simulink model "Sim_Forcing_003h_expe_infra5_full_control2"  (Simulink 7.4)
settings: Solver=FixedStepDiscrete  StartTime=0.0  StopTime=inf  FixedStep=0.004  RelTol=1e-3
undefined symbols (not defined in the file or in its folder): DiscIntNeverNeededParam
libraries: simulink x43, gt_rt_lib x22, xpcutilitieslib x4, xpclib x2, dspswit3 x1
(part 2 of 4)

== system Sim_Forcing_003h_expe_infra5_full_control2/Breaking_Control 20/07/15/Smooth Displacement Second-Order Filter, zeta 0.8 ==
  Step IN Reset on  either : Inport
  T : Inport  Port=2  OutDataType=fixdt(1, 16)  OutScaling=2^0
  (zeta*T_transfer)/pi : Gain  Gain=0.8/pi  ParameterDataType=fixdt(1, 16)  ParameterScaling=2^0  OutDataType=fixdt(1, 16)  OutScaling=2^0
  4*zeta*pi : Gain  Gain=3.2*pi  ParameterDataType=fixdt(1, 16)  ParameterScaling=2^0  OutDataType=fixdt(1, 16)  OutScaling=2^0
  4*zeta*pi/T_transfer /s : DiscreteIntegrator  gainval=1  ExternalReset=either  InitialConditionSource=external  SampleTime=0.004  OutDataType=fixdt(1, 16)  OutScaling=2^0  ICPrevOutput=DiscIntNeverNeededParam  ICPrevScaledInput=DiscIntNeverNeededParam
  Discrete Derivative : simulink/Discrete/Discrete Derivative  SystemSampleTime=-1  gainval=1.0  ICPrevScaledInput=0.0  OutMin=[]  OutMax=[]  OutDataType=fixdt(1, 16)  OutScaling=2^-10  DoSatur=off
  Divide : Product  Inputs=*/  OutDataType=fixdt(1, 16)  OutScaling=2^-10
  Divide1 : Product  Inputs=*/  OutDataType=fixdt(1, 16)  OutScaling=2^-10
  For saving position  and velocity until after switchover : UnitDelay  SampleTime=-1
  Product : Product  OutDataType=fixdt(1, 16)  OutScaling=2^0  RndMeth=Zero
  Sum1 : Sum  Inputs=|+-  OutDataType=fixdt(1, 16)  OutScaling=2^0
  Sum2 : Sum  Inputs=-+|  OutDataType=fixdt(1, 16)  OutScaling=2^0
  pi/(zeta*T_transfer)/s : DiscreteIntegrator  gainval=1  ExternalReset=either  InitialConditionSource=external  SampleTime=0.004  OutDataType=fixdt(1, 16)  OutScaling=2^0  ICPrevOutput=DiscIntNeverNeededParam  ICPrevScaledInput=DiscIntNeverNeededParam
  pi/zeta : Gain  Gain=pi/0.8  ParameterDataType=fixdt(1, 16)  ParameterScaling=2^0  OutDataType=fixdt(1, 16)  OutScaling=2^0
  Out : Outport
  wires:
  Discrete Derivative/1 -> Product/2
  Product/1 -> (zeta*T_transfer)/pi/1
  Divide/1 -> 4*zeta*pi/1
  Divide1/1 -> pi/zeta/1
  pi/zeta/1 -> pi/(zeta*T_transfer)/s/1
  pi/(zeta*T_transfer)/s/1 -> Sum2/1, Out/1, For saving position  and velocity until after switchover/1
  4*zeta*pi/T_transfer /s/1 -> Divide1/1, Sum1/2
  Sum1/1 -> Divide/1
  4*zeta*pi/1 -> 4*zeta*pi/T_transfer /s/1
  T/1 -> [T]
  Step IN Reset on  either/1 -> [Step], Sum2/2
  [Step] -> 4*zeta*pi/T_transfer /s/2
  [Step] -> pi/(zeta*T_transfer)/s/2
  [T] -> Divide/2
  For saving position  and velocity until after switchover/1 -> Discrete Derivative/1, pi/(zeta*T_transfer)/s/3
  [T] -> Product/1
  (zeta*T_transfer)/pi/1 -> 4*zeta*pi/T_transfer /s/3
  [T] -> Divide1/2
  Sum2/1 -> Sum1/1

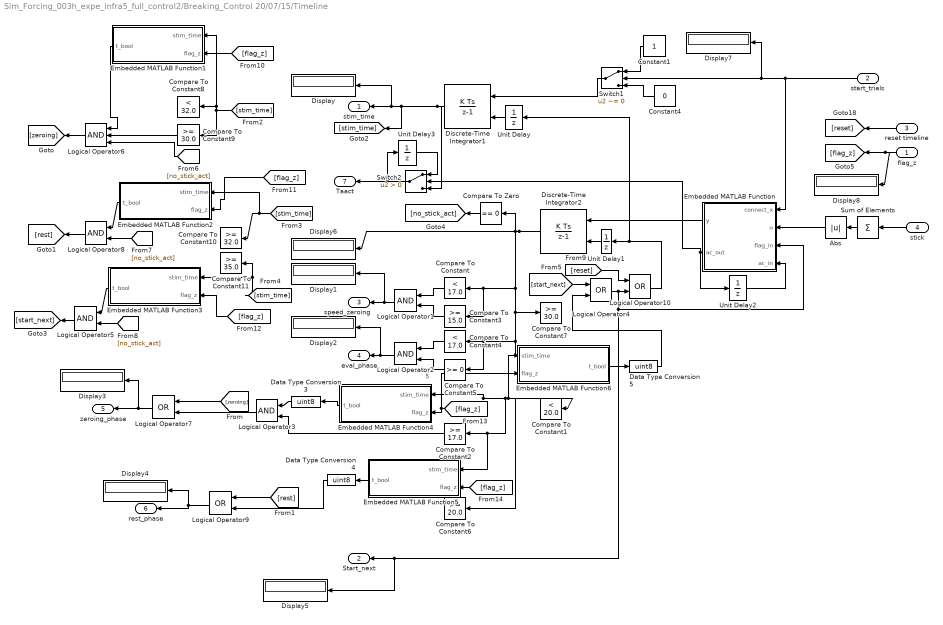
== system Sim_Forcing_003h_expe_infra5_full_control2/Breaking_Control 20/07/15/Timeline ==
  note: 5
  flag_z : Inport  PortDimensions=1
  start_trials : Inport  Port=2  PortDimensions=1
  reset timeline : Inport  Port=3  PortDimensions=1
  stick : Inport  Port=4
  Abs : Abs  OutDataType=fixdt(1, 16)  OutScaling=2^0
  Compare To Constant : simulink/Logic and Bit Operations/Compare To Constant  SystemSampleTime=-1  relop=<  const=17.0  LogicOutDataTypeMode=uint8
  Compare To Constant1 : simulink/Logic and Bit Operations/Compare To Constant  SystemSampleTime=-1  relop=<  const=20.0  LogicOutDataTypeMode=uint8
  Compare To Constant10 : simulink/Logic and Bit Operations/Compare To Constant  SystemSampleTime=-1  relop=>=  const=32.0  LogicOutDataTypeMode=uint8
  Compare To Constant11 : simulink/Logic and Bit Operations/Compare To Constant  SystemSampleTime=-1  relop=>=  const=35.0  LogicOutDataTypeMode=uint8
  Compare To Constant2 : simulink/Logic and Bit Operations/Compare To Constant  SystemSampleTime=-1  relop=>=  const=17.0  LogicOutDataTypeMode=uint8
  Compare To Constant3 : simulink/Logic and Bit Operations/Compare To Constant  SystemSampleTime=-1  relop=>=  const=15.0  LogicOutDataTypeMode=uint8
  Compare To Constant4 : simulink/Logic and Bit Operations/Compare To Constant  SystemSampleTime=-1  relop=<  const=17.0  LogicOutDataTypeMode=uint8
  Compare To Constant5 : simulink/Logic and Bit Operations/Compare To Constant  SystemSampleTime=-1  relop=>=  const=0  LogicOutDataTypeMode=uint8
  Compare To Constant6 : simulink/Logic and Bit Operations/Compare To Constant  SystemSampleTime=-1  relop=>=  const=20.0  LogicOutDataTypeMode=uint8
  Compare To Constant7 : simulink/Logic and Bit Operations/Compare To Constant  SystemSampleTime=-1  relop=>=  const=30.0  LogicOutDataTypeMode=uint8
  Compare To Constant8 : simulink/Logic and Bit Operations/Compare To Constant  SystemSampleTime=-1  relop=<  const=32.0  LogicOutDataTypeMode=uint8
  Compare To Constant9 : simulink/Logic and Bit Operations/Compare To Constant  SystemSampleTime=-1  relop=>=  const=30.0  LogicOutDataTypeMode=uint8
  Compare To Zero : simulink/Logic and Bit Operations/Compare To Zero  SystemSampleTime=-1  relop===  LogicOutDataTypeMode=uint8
  Constant1 : Constant  OutDataType=fixdt(1, 16)  OutScaling=2^0
  Constant4 : Constant  Value=0  OutDataType=fixdt(1, 16)  OutScaling=2^0
  Data Type Conversion3 : DataTypeConversion  OutDataTypeMode=uint8  OutDataType=fixdt(1, 16)  OutScaling=2^0  OutDataTypeStr=uint8
  Data Type Conversion4 : DataTypeConversion  OutDataTypeMode=uint8  OutDataType=fixdt(1, 16)  OutScaling=2^0  OutDataTypeStr=uint8
  Data Type Conversion5 : DataTypeConversion  OutDataTypeMode=uint8  OutDataType=fixdt(1, 16)  OutScaling=2^0  OutDataTypeStr=uint8
  Discrete-Time Integrator1 : DiscreteIntegrator  ExternalReset=rising  SampleTime=0.004  LimitOutput=on  UpperSaturationLimit=60  LowerSaturationLimit=0  ICPrevOutput=DiscIntNeverNeededParam  ICPrevScaledInput=DiscIntNeverNeededParam
  Discrete-Time Integrator2 : DiscreteIntegrator  ExternalReset=rising  SampleTime=0.004  LimitOutput=on  UpperSaturationLimit=40  LowerSaturationLimit=0  ICPrevOutput=DiscIntNeverNeededParam  ICPrevScaledInput=DiscIntNeverNeededParam
  Display{,1..8} (9 alike) : Display
  Embedded MATLAB Function : Stateflow chart
  Embedded MATLAB Function1 : Stateflow chart
  Embedded MATLAB Function2 : Stateflow chart
  Embedded MATLAB Function3 : Stateflow chart
  Embedded MATLAB Function4 : Stateflow chart
  Embedded MATLAB Function5 : Stateflow chart
  Embedded MATLAB Function6 : Stateflow chart
  Logical Operator{1..3,5,8} (5 alike) : Logic  AllPortsSameDT=off  OutDataTypeMode=boolean  LogicDataType=fixdt(0, 8)  OutDataTypeStr=boolean
  Logical Operator{4,7,9..10} (4 alike) : Logic  Operator=OR  AllPortsSameDT=off  OutDataTypeMode=boolean  LogicDataType=fixdt(0, 8)  OutDataTypeStr=boolean
  Logical Operator6 : Logic  Inputs=3  AllPortsSameDT=off  OutDataTypeMode=boolean  LogicDataType=fixdt(0, 8)  OutDataTypeStr=boolean
  Sum of Elements : Sum  Inputs=+  OutDataType=fixdt(1, 16)  OutScaling=2^-10
  Switch1 : Switch  Criteria=u2 ~= 0  Threshold=0.2  OutDataType=fixdt(1, 16)  OutScaling=2^0
  Switch2 : Switch  Criteria=u2 > Threshold  OutDataType=fixdt(1, 16)  OutScaling=2^0
  Unit Delay{,1..3} (4 alike) : UnitDelay  SampleTime=-1
  stim_time : Outport  OutDataType=fixdt(1, 16)  OutScaling=2^0
  Start_next : Outport  Port=2  OutDataType=fixdt(1, 16)  OutScaling=2^0
  speed_zeroing : Outport  Port=3  OutDataType=fixdt(1, 16)  OutScaling=2^0
  eval_phase : Outport  Port=4  OutDataType=fixdt(1, 16)  OutScaling=2^0
  zeroing_phase : Outport  Port=5  OutDataType=fixdt(1, 16)  OutScaling=2^0
  rest_phase : Outport  Port=6  OutDataType=fixdt(1, 16)  OutScaling=2^0
  Taact : Outport  Port=7  OutDataType=fixdt(1, 16)  OutScaling=2^0
  wires:
  Discrete-Time Integrator1/1 -> stim_time/1, Display/1, [stim_time], Switch2/3
  Embedded MATLAB Function/1(y) -> Discrete-Time Integrator2/1
  Discrete-Time Integrator2/1 -> Compare To Constant/1, Compare To Constant3/1, Compare To Constant4/1, Compare To Constant5/1, Compare To Constant1/1, Embedded MATLAB Function4/1(stim_time), Compare To Constant2/1, Embedded MATLAB Function5/1(stim_time), Compare To Constant6/1, Embedded MATLAB Function6/1(stim_time), Compare To Constant7/1, Display6/1, Compare To Zero/1
  Compare To Constant/1 -> Logical Operator1/1
  Compare To Constant3/1 -> Logical Operator1/2
  Logical Operator1/1 -> speed_zeroing/1, Display1/1
  Compare To Constant4/1 -> Logical Operator2/1
  Compare To Constant5/1 -> Logical Operator2/2
  Logical Operator2/1 -> eval_phase/1, Display2/1
  Compare To Constant2/1 -> Logical Operator3/2
  Logical Operator3/1 -> Logical Operator7/2
  Logical Operator4/1 -> Start_next/1, Display5/1, Embedded MATLAB Function/3(flag_in), Logical Operator10/2
  Constant1/1 -> Switch1/1
  Switch1/1 -> Discrete-Time Integrator1/1
  start_trials/1 -> Switch1/2, Display7/1, Embedded MATLAB Function/1(connect_x)
  Constant4/1 -> Switch1/3
  stick/1 -> Sum of Elements/1
  Unit Delay/1 -> Discrete-Time Integrator1/2
  Unit Delay1/1 -> Discrete-Time Integrator2/2
  Sum of Elements/1 -> Abs/1
  Abs/1 -> Embedded MATLAB Function/2(u)
  Embedded MATLAB Function/2(ac_out) -> Unit Delay2/1, Switch2/2
  Unit Delay2/1 -> Embedded MATLAB Function/4(ac_in)
  Compare To Constant9/1 -> Logical Operator6/2
  Logical Operator7/1 -> zeroing_phase/1, Display3/1
  Logical Operator9/1 -> rest_phase/1, Display4/1
  Logical Operator6/1 -> [zeroing]
  [zeroing] -> Logical Operator7/1
  Logical Operator8/1 -> [rest]
  [rest] -> Logical Operator9/1
  [stim_time] -> Compare To Constant9/1, Compare To Constant8/1, Embedded MATLAB Function1/1(stim_time)
  [stim_time] -> Compare To Constant10/1, Embedded MATLAB Function2/1(stim_time)
  [stim_time] -> Compare To Constant11/1, Embedded MATLAB Function3/1(stim_time)
  Logical Operator5/1 -> [start_next]
  [start_next] -> Logical Operator4/1
  Compare To Zero/1 -> [no_stick_act]
  [no_stick_act] -> Logical Operator6/3
  [no_stick_act] -> Logical Operator8/2
  [no_stick_act] -> Logical Operator5/2
  reset timeline/1 -> [reset]
  flag_z/1 -> [flag_z], Display8/1
  [flag_z] -> Embedded MATLAB Function4/2(flag_z), Embedded MATLAB Function6/2(flag_z)
  [flag_z] -> Embedded MATLAB Function5/2(flag_z)
  Embedded MATLAB Function4/1(t_bool) -> Data Type Conversion3/1
  Data Type Conversion3/1 -> Logical Operator3/1
  Embedded MATLAB Function5/1(t_bool) -> Data Type Conversion4/1
  Data Type Conversion4/1 -> Logical Operator9/2
  Embedded MATLAB Function6/1(t_bool) -> Data Type Conversion5/1
  Data Type Conversion5/1 -> Logical Operator4/2
  Switch2/1 -> Taact/1, Unit Delay3/1
  Unit Delay3/1 -> Switch2/1
  [reset] -> Logical Operator10/1
  Logical Operator10/1 -> Unit Delay1/1, Unit Delay/1
  [flag_z] -> Embedded MATLAB Function1/2(flag_z)
  Embedded MATLAB Function1/1(t_bool) -> Logical Operator6/1
  Embedded MATLAB Function2/1(t_bool) -> Logical Operator8/1
  [flag_z] -> Embedded MATLAB Function2/2(flag_z)
  Embedded MATLAB Function3/1(t_bool) -> Logical Operator5/1
  [flag_z] -> Embedded MATLAB Function3/2(flag_z)

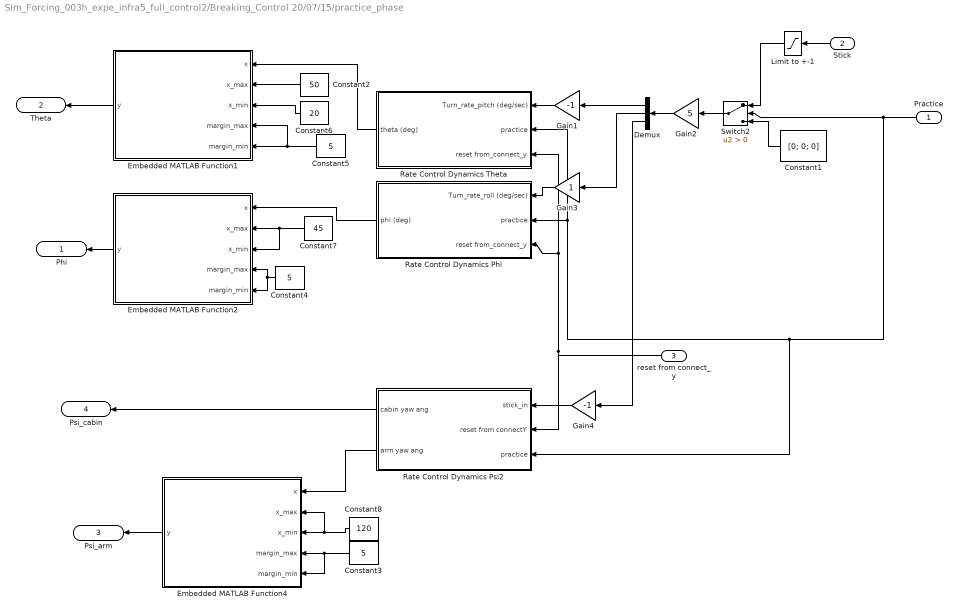
== system Sim_Forcing_003h_expe_infra5_full_control2/Breaking_Control 20/07/15/practice_phase ==
  Practice : Inport  OutDataType=fixdt(1, 16)  OutScaling=2^0
  Stick : Inport  Port=2
  reset from connect_y : Inport  Port=3
  Constant1 : Constant  Value=[0; 0; 0]  OutDataType=fixdt(1, 16)  OutScaling=2^0
  Constant2 : Constant  Value=50  OutDataType=fixdt(1, 16)  OutScaling=2^0
  Constant3 : Constant  Value=5  OutDataType=fixdt(1, 16)  OutScaling=2^0
  Constant4 : Constant  Value=5  OutDataType=fixdt(1, 16)  OutScaling=2^0
  Constant5 : Constant  Value=5  OutDataType=fixdt(1, 16)  OutScaling=2^0
  Constant6 : Constant  Value=20  OutDataType=fixdt(1, 16)  OutScaling=2^0
  Constant7 : Constant  Value=45  OutDataType=fixdt(1, 16)  OutScaling=2^0
  Constant8 : Constant  Value=120  OutDataType=fixdt(1, 16)  OutScaling=2^0
  Demux : Demux  Outputs=3
  Embedded MATLAB Function1 : Stateflow chart
  Embedded MATLAB Function2 : Stateflow chart
  Embedded MATLAB Function4 : Stateflow chart
  Gain1 : Gain  Gain=-1  ParameterDataType=fixdt(1, 16)  ParameterScaling=2^0  OutDataType=fixdt(1, 16)  OutScaling=2^0
  Gain2 : Gain  Gain=5  ParameterDataType=fixdt(1, 16)  ParameterScaling=2^0  OutDataType=fixdt(1, 16)  OutScaling=2^0
  Gain3 : Gain  ParameterDataType=fixdt(1, 16)  ParameterScaling=2^0  OutDataType=fixdt(1, 16)  OutScaling=2^0
  Gain4 : Gain  Gain=-1  ParameterDataType=fixdt(1, 16)  ParameterScaling=2^0  OutDataType=fixdt(1, 16)  OutScaling=2^0
  Limit to +-1 : Saturate  UpperLimit=1  LowerLimit=-1  OutDataType=fixdt(1, 16)  OutScaling=2^0
  Rate Control Dynamics Phi : Subsystem
  Rate Control Dynamics Psi2 : Subsystem
  Rate Control Dynamics Theta : Subsystem
  Switch2 : Switch  Criteria=u2 > Threshold  OutDataType=fixdt(1, 16)  OutScaling=2^0
  Phi : Outport
  Theta : Outport  Port=2
  Psi_arm : Outport  Port=3
  Psi_cabin : Outport  Port=4
  wires:
  Gain2/1 -> Demux/1
  Demux/1 -> Gain1/1
  Demux/2 -> Gain3/1
  Gain1/1 -> Rate Control Dynamics Theta/1(Turn_rate_pitch (deg/sec))
  Switch2/1 -> Gain2/1
  Stick/1 -> Limit to +-1/1
  reset from connect_y/1 -> Rate Control Dynamics Phi/3(reset from_connect_y), Rate Control Dynamics Theta/3(reset from_connect_y), Rate Control Dynamics Psi2/2(reset from connectY)
  Gain3/1 -> Rate Control Dynamics Phi/1(Turn_rate_roll (deg/sec))
  Demux/3 -> Gain4/1
  Practice/1 -> Switch2/2, Rate Control Dynamics Phi/2(practice), Rate Control Dynamics Theta/2(practice), Rate Control Dynamics Psi2/3(practice)
  Limit to +-1/1 -> Switch2/1
  Constant1/1 -> Switch2/3
  Gain4/1 -> Rate Control Dynamics Psi2/1(stick_in)
  Rate Control Dynamics Psi2/1(cabin yaw ang) -> Psi_cabin/1
  Embedded MATLAB Function1/1(y) -> Theta/1
  Constant7/1 -> Embedded MATLAB Function2/2(x_max), Embedded MATLAB Function2/3(x_min)
  Rate Control Dynamics Phi/1(phi (deg)) -> Embedded MATLAB Function2/1(x)
  Embedded MATLAB Function2/1(y) -> Phi/1
  Constant3/1 -> Embedded MATLAB Function4/4(margin_max), Embedded MATLAB Function4/5(margin_min)
  Constant8/1 -> Embedded MATLAB Function4/3(x_min), Embedded MATLAB Function4/2(x_max)
  Embedded MATLAB Function4/1(y) -> Psi_arm/1
  Constant4/1 -> Embedded MATLAB Function2/4(margin_max), Embedded MATLAB Function2/5(margin_min)
  Constant5/1 -> Embedded MATLAB Function1/4(margin_max), Embedded MATLAB Function1/5(margin_min)
  Constant6/1 -> Embedded MATLAB Function1/3(x_min)
  Constant2/1 -> Embedded MATLAB Function1/2(x_max)
  Rate Control Dynamics Theta/1(theta (deg)) -> Embedded MATLAB Function1/1(x)
  Rate Control Dynamics Psi2/2(arm yaw ang) -> Embedded MATLAB Function4/1(x)

== system Sim_Forcing_003h_expe_infra5_full_control2/Breaking_Control 20/07/15/select_ang_speed ==
  Count : Inport  OutDataType=fixdt(1, 16)  OutScaling=2^0
  eval_phase : Inport  Port=2  OutDataType=fixdt(1, 16)  OutScaling=2^0
  Constant : Constant  Value=[0 0 0]  OutDataType=fixdt(1, 16)  OutScaling=2^0
  Embedded MATLAB Function2 : Stateflow chart
  Switch : Switch  Criteria=u2 ~= 0  OutDataType=fixdt(1, 16)  OutScaling=2^0
  Unit Delay : UnitDelay  SampleTime=-1
  Target_ang_speed : Outport
  mask : Outport  Port=2
  vis_cond : Outport  Port=3
  flag_out : Outport  Port=4
  eof : Outport  Port=5
  wires:
  Count/1 -> Embedded MATLAB Function2/1(count)
  eval_phase/1 -> Switch/2
  Embedded MATLAB Function2/1(target_ang_speed) -> Switch/3, Target_ang_speed/1
  Constant/1 -> Switch/1
  Embedded MATLAB Function2/2(mask) -> mask/1
  Embedded MATLAB Function2/3(vis_cond) -> vis_cond/1
  Embedded MATLAB Function2/4(flag_out) -> flag_out/1
  Embedded MATLAB Function2/5(endOffile_out) -> Unit Delay/1, eof/1
  Unit Delay/1 -> Embedded MATLAB Function2/2(endOffile_in)

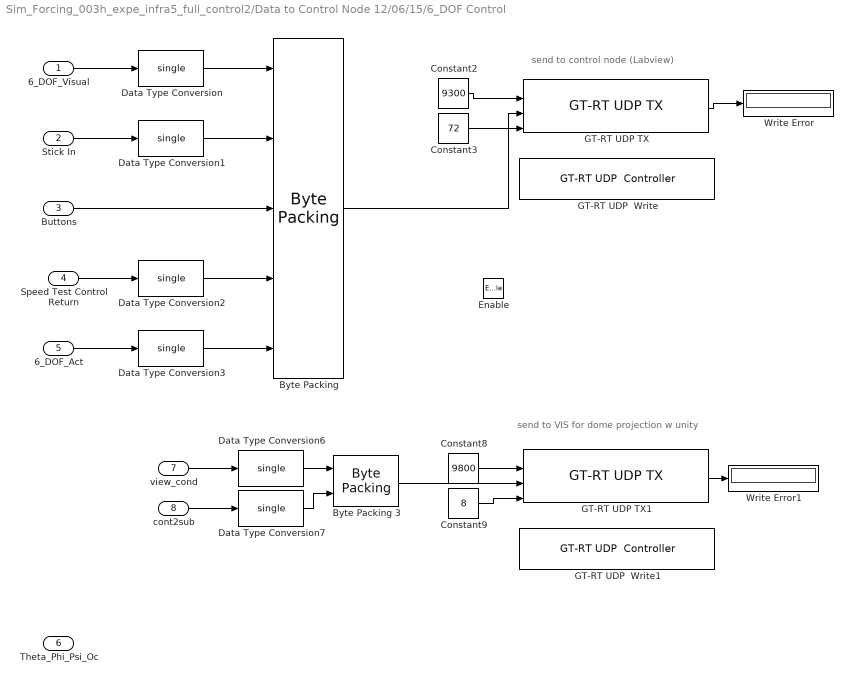
== system Sim_Forcing_003h_expe_infra5_full_control2/Data to Control Node 12/06/15/6_DOF Control ==
  note: send to control node (Labview)
  note: send to VIS for dome projection w unity
  6_DOF_Visual : Inport
  Stick In : Inport  Port=2
  Buttons : Inport  Port=3
  Speed Test Control Return : Inport  Port=4
  6_DOF_Act : Inport  Port=5
  Theta_Phi_Psi_Oc : Inport  Port=6
  view_cond : Inport  Port=7
  cont2sub : Inport  Port=8
  Enable : EnablePort
  "Byte Packing " : xpcutilitieslib/Byte Packing   MaskPackedDataType=uint8  MaskUnpackedDataTypes={'single','single','uint8','single','single'}  MaskAlignment=1
  Byte Packing 3 : xpcutilitieslib/Byte Packing   MaskPackedDataType=uint8  MaskUnpackedDataTypes={'single','single'}  MaskAlignment=1
  Constant2 : Constant  Value=9300  OutDataTypeMode=uint16  OutDataType=fixdt(1, 16)  OutScaling=2^0  OutDataTypeStr=uint16
  Constant3 : Constant  Value=72  OutDataTypeMode=uint32  OutDataType=fixdt(1, 16)  OutScaling=2^0  OutDataTypeStr=uint32
  Constant8 : Constant  Value=9800  OutDataTypeMode=uint16  OutDataType=fixdt(1, 16)  OutScaling=2^0  OutDataTypeStr=uint16
  Constant9 : Constant  Value=8  OutDataTypeMode=uint32  OutDataType=fixdt(1, 16)  OutScaling=2^0  OutDataTypeStr=uint32
  Data Type Conversion{,1..3,6..7} (6 alike) : DataTypeConversion  OutDataTypeMode=single  OutDataType=fixdt(1, 16)  OutScaling=2^0  OutDataTypeStr=single
  GT-RT UDP  Write : gt_rt_lib/GT-RT UDP  Controller  uri='gtp://localhost/udp?port=9300'
  GT-RT UDP  Write1 : gt_rt_lib/GT-RT UDP  Controller  uri='gtp://localhost/udp?port=9800'
  GT-RT UDP TX : gt_rt_lib/GT-RT UDP TX  uri='gtp://localhost/udp?port=9300'  hostname='192.168.102.75'
  GT-RT UDP TX1 : gt_rt_lib/GT-RT UDP TX  uri='gtp://localhost/udp?port=9800'  hostname='192.168.102.13'
  Write Error : Display
  Write Error1 : Display
  wires:
  Constant2/1 -> GT-RT UDP TX/2
  Constant3/1 -> GT-RT UDP TX/4
  GT-RT UDP TX/1 -> Write Error/1
  Data Type Conversion/1 -> "Byte Packing "/1
  "Byte Packing "/1 -> GT-RT UDP TX/3
  Stick In/1 -> Data Type Conversion1/1
  Data Type Conversion1/1 -> "Byte Packing "/2
  Buttons/1 -> "Byte Packing "/3
  Speed Test Control Return/1 -> Data Type Conversion2/1
  Data Type Conversion2/1 -> "Byte Packing "/4
  6_DOF_Act/1 -> Data Type Conversion3/1
  Data Type Conversion3/1 -> "Byte Packing "/5
  GT-RT UDP TX1/1 -> Write Error1/1
  6_DOF_Visual/1 -> Data Type Conversion/1
  Constant8/1 -> GT-RT UDP TX1/2
  Constant9/1 -> GT-RT UDP TX1/4
  Byte Packing 3/1 -> GT-RT UDP TX1/3
  view_cond/1 -> Data Type Conversion6/1
  Data Type Conversion6/1 -> Byte Packing 3/1
  cont2sub/1 -> Data Type Conversion7/1
  Data Type Conversion7/1 -> Byte Packing 3/2

== system Sim_Forcing_003h_expe_infra5_full_control2/Data to Control Node 12/06/15/Interaction device from VIS (Stick)  ==
  Display2 : Display
  Display4 : Display
  Display5 : Display
  Error : Display
  GT-RT UDP  Read : gt_rt_lib/GT-RT UDP  Controller  uri='gtp://localhost/udp?port=9600'
  GT-RT UDP RX : gt_rt_lib/GT-RT UDP RX  uri='gtp://localhost/udp?port=9600'  receive_buffer_size=28  timeout=0  sample_time=0.004
  Terminator : Terminator
  Unpack : xpclib/UDP/Unpack  dimensions={3,8,1,1}  datatypes={'single','uint8','single','single'}  byteAlign=1
  Stick Out : Outport  OutDataType=fixdt(1, 16)  OutScaling=2^0
  Buttons : Outport  Port=2  OutDataType=fixdt(1, 16)  OutScaling=2^0
  Speed_Test_VIS_Send : Outport  Port=3  OutDataType=fixdt(1, 16)  OutScaling=2^0
  for_delay_calc : Outport  Port=4  OutDataType=fixdt(1, 16)  OutScaling=2^0
  wires:
  GT-RT UDP RX/2 -> Display2/1
  GT-RT UDP RX/6 -> Error/1
  GT-RT UDP RX/5 -> Display4/1
  GT-RT UDP RX/4 -> Display5/1
  GT-RT UDP RX/1 -> Unpack/1
  GT-RT UDP RX/3 -> Terminator/1
  Unpack/1 -> Stick Out/1
  Unpack/2 -> Buttons/1
  Unpack/3 -> Speed_Test_VIS_Send/1
  Unpack/4 -> for_delay_calc/1

== system Sim_Forcing_003h_expe_infra5_full_control2/Handshake CAN/If Action Subsystem ==
  Action Port : ActionPort
  GT-RT CAN TX : gt_rt_lib/GT-RT CAN TX  uri='gt_rt_dev://localhost/dev/can0#0'  mff=MFF_11_DAT
  TX CAN ID1 : Constant  Value=hex2dec('100')  OutDataTypeMode=uint32  OutDataType=sfix(16)  OutScaling=2^0  OutDataTypeStr=uint32
  TX Data : Constant  OutDataTypeMode=uint8  OutDataType=sfix(16)  OutScaling=2^0  OutDataTypeStr=uint8
  wires:
  TX CAN ID1/1 -> GT-RT CAN TX/1
  TX Data/1 -> GT-RT CAN TX/2

== system Sim_Forcing_003h_expe_infra5_full_control2/Handshake CAN/If Action Subsystem1 ==
  Action Port : ActionPort  ActionType=then
  GT-RT CAN TX : gt_rt_lib/GT-RT CAN TX  uri='gt_rt_dev://localhost/dev/can0#0'  mff=MFF_11_DAT
  TX CAN ID1 : Constant  Value=hex2dec('100')  OutDataTypeMode=uint32  OutDataType=sfix(16)  OutScaling=2^0  OutDataTypeStr=uint32
  TX Data : Constant  OutDataTypeMode=uint8  OutDataType=sfix(16)  OutScaling=2^0  OutDataTypeStr=uint8
  wires:
  TX CAN ID1/1 -> GT-RT CAN TX/1
  TX Data/1 -> GT-RT CAN TX/2

== system Sim_Forcing_003h_expe_infra5_full_control2/Joint Controller (May 7, 2015)1/Forward Kinematics ==
  J_ANG_ACT : Inport
  Data Type Conversion4 : DataTypeConversion  OutDataTypeMode=double  OutDataType=fixdt(1, 16)  OutScaling=2^0  OutDataTypeStr=double
  Demux1 : Demux  Outputs=[3,1,1,1]
  Embedded MATLAB Function : Stateflow chart
  KUKA2NED : Subsystem
  Mux : Mux  Inputs=3
  6-DOF_ACT : Outport
  roll_pitch_yaw_act : Outport  Port=2
  wires:
  KUKA2NED/1(NED) -> Embedded MATLAB Function/1(vec)
  Embedded MATLAB Function/1(out) -> 6-DOF_ACT/1, Data Type Conversion4/1
  J_ANG_ACT/1 -> KUKA2NED/1(KUKA)
  Demux1/3 -> Mux/2
  Demux1/2 -> Mux/1
  Mux/1 -> roll_pitch_yaw_act/1
  Data Type Conversion4/1 -> Demux1/1
  Demux1/4 -> Mux/3

== system Sim_Forcing_003h_expe_infra5_full_control2/Joint Controller (May 7, 2015)1/Increments ==
  J_ANG : Inport
  Sum6 : Sum  Inputs=|+-  OutDataType=fixdt(1, 16)  OutScaling=2^0
  Unit Delay6 : UnitDelay  X0=[0 50 -68 0 18 0]'  SampleTime=-1
  J_ANG_INC : Outport
  wires:
  Unit Delay6/1 -> Sum6/2
  J_ANG/1 -> Unit Delay6/1, Sum6/1
  Sum6/1 -> J_ANG_INC/1

== system Sim_Forcing_003h_expe_infra5_full_control2/Joint Controller (May 7, 2015)1/Inverse Kinematics May 6, 2015 ==
  note: Delay of 0.004s to initialize the currect step with the value of J_ANG of the previous loop
  6-DOF : Inport  OutDataType=fixdt(1, 16)  OutScaling=2^0
  Activate_full_inverse : Inport  Port=2  OutDataType=fixdt(1, 16)  OutScaling=2^0
  6_DOF_ACT : Inport  Port=3  OutDataType=fixdt(1, 16)  OutScaling=2^0
  Constant : Constant  OutDataType=fixdt(1, 16)  OutScaling=2^0
  Demux : Demux  Outputs=[6 1]
  Ground : Ground
  Inverse Kinematics : Subsystem
  Mux : Mux  Inputs=2
  NED2KUKA : Subsystem
  Scope1 : Scope
      settings: YMin=-50  YMax=70  SaveName=ScopeData4
  Simplified Inverse Kinematics : Subsystem
  Starting Joint Angles KUKA : Constant  Value=[0 -50 68 0 -18 15.89]'  OutDataType=fixdt(1, 16)  OutScaling=2^0
  Starting Joint Angles NED : Constant  Value=[0 50 -68 0 18 0]'  OutDataType=fixdt(1, 16)  OutScaling=2^0
  Switch : Switch  Criteria=u2 > Threshold  OutDataType=fixdt(1, 16)  OutScaling=2^0
  Switch1 : Switch  Criteria=u2 > Threshold  OutDataType=fixdt(1, 16)  OutScaling=2^0
  Unit Delay : UnitDelay  X0=[0 50 -68 0 18 0]'  SampleTime=-1
  J_ANG : Outport  OutDataType=fixdt(1, 16)  OutScaling=2^0
  N : Outport  Port=2  OutDataType=fixdt(1, 16)  OutScaling=2^0
  wires:
  NED2KUKA/1(KUKA) -> Scope1/1, J_ANG/1
  6-DOF/1 -> Mux/1
  Unit Delay/1 -> Mux/2
  Demux/1 -> NED2KUKA/1(NED), Unit Delay/1
  Demux/2 -> N/1
  Simplified Inverse Kinematics/1(out) -> Switch/1
  Inverse Kinematics/1(out) -> Switch/3
  Switch/1 -> Demux/1
  Mux/1 -> Inverse Kinematics/1(vec), Simplified Inverse Kinematics/2(vec)
  Activate_full_inverse/1 -> Inverse Kinematics/2(Activate full inverse), Switch1/2
  Ground/1 -> Switch1/1
  Switch1/1 -> Simplified Inverse Kinematics/1(activate simplified), Switch/2
  Constant/1 -> Switch1/3
  6_DOF_ACT/1 -> Inverse Kinematics/3(6_DOF_ACT)

== system Sim_Forcing_003h_expe_infra5_full_control2/Joint Controller (May 7, 2015)1/Subtract psi offset ==
  Psi_Offset : Inport
  J_ANG_ACT : Inport  Port=2
  Data Type Conversion : DataTypeConversion  OutDataTypeMode=double  OutDataType=fixdt(1, 16)  OutScaling=2^0  OutDataTypeStr=double
  Demux1 : Demux  Outputs=[1,5]
  Mux1 : Mux  Inputs=[1,5]
  Sum3 : Sum  Inputs=-+|  OutDataType=fixdt(1, 16)  OutScaling=2^0
  out : Outport
  wires:
  Demux1/1 -> Sum3/2
  Sum3/1 -> Mux1/1
  Demux1/2 -> Mux1/2
  J_ANG_ACT/1 -> Data Type Conversion/1
  Mux1/1 -> out/1
  Data Type Conversion/1 -> Demux1/1
  Psi_Offset/1 -> Sum3/1

== system Sim_Forcing_003h_expe_infra5_full_control2/BEC (May 7, 2015)/CAN Receive/Convert 4*uni8 to int ==
  byte0 : Inport
  byte1 : Inport  Port=2
  byte2 : Inport  Port=3
  byte3 : Inport  Port=4
  Add : Sum  Inputs=++++  OutDataTypeMode=int32  OutDataType=fixdt(1, 16)  OutScaling=2^-10  OutDataTypeStr=int32
  Gain2 : Gain  Gain=256  ParameterDataType=fixdt(1, 16)  ParameterScaling=2^0  OutDataType=fixdt(1, 16)  OutScaling=2^0
  Gain3 : Gain  Gain=2^16  ParameterDataType=fixdt(1, 16)  ParameterScaling=2^0  OutDataType=fixdt(1, 16)  OutScaling=2^0
  Gain4 : Gain  Gain=2^24  ParameterDataType=fixdt(1, 16)  ParameterScaling=2^0  OutDataType=fixdt(1, 16)  OutScaling=2^0
  int : Outport
  wires:
  Gain2/1 -> Add/2
  Gain3/1 -> Add/3
  byte0/1 -> Add/1
  Add/1 -> int/1
  byte1/1 -> Gain2/1
  byte2/1 -> Gain3/1
  byte3/1 -> Gain4/1
  Gain4/1 -> Add/4

== system Sim_Forcing_003h_expe_infra5_full_control2/BEC (May 7, 2015)/CAN Receive/Convert 4*uni8 to int1 ==
  byte0 : Inport
  byte1 : Inport  Port=2
  byte2 : Inport  Port=3
  byte3 : Inport  Port=4
  Add : Sum  Inputs=++++  OutDataTypeMode=int32  OutDataType=fixdt(1, 16)  OutScaling=2^-10  OutDataTypeStr=int32
  Gain2 : Gain  Gain=256  ParameterDataType=fixdt(1, 16)  ParameterScaling=2^0  OutDataType=fixdt(1, 16)  OutScaling=2^0
  Gain3 : Gain  Gain=2^16  ParameterDataType=fixdt(1, 16)  ParameterScaling=2^0  OutDataType=fixdt(1, 16)  OutScaling=2^0
  Gain4 : Gain  Gain=2^24  ParameterDataType=fixdt(1, 16)  ParameterScaling=2^0  OutDataType=fixdt(1, 16)  OutScaling=2^0
  int : Outport
  wires:
  Gain4/1 -> Add/4
  byte3/1 -> Gain4/1
  byte2/1 -> Gain3/1
  byte1/1 -> Gain2/1
  Add/1 -> int/1
  byte0/1 -> Add/1
  Gain3/1 -> Add/3
  Gain2/1 -> Add/2

== system Sim_Forcing_003h_expe_infra5_full_control2/BEC (May 7, 2015)/CAN Receive/Convert 4*uni8 to int2 ==
  byte0 : Inport
  byte1 : Inport  Port=2
  byte2 : Inport  Port=3
  byte3 : Inport  Port=4
  Add : Sum  Inputs=++++  OutDataTypeMode=int32  OutDataType=fixdt(1, 16)  OutScaling=2^-10  OutDataTypeStr=int32
  Gain2 : Gain  Gain=256  ParameterDataType=fixdt(1, 16)  ParameterScaling=2^0  OutDataType=fixdt(1, 16)  OutScaling=2^0
  Gain3 : Gain  Gain=2^16  ParameterDataType=fixdt(1, 16)  ParameterScaling=2^0  OutDataType=fixdt(1, 16)  OutScaling=2^0
  Gain4 : Gain  Gain=2^24  ParameterDataType=fixdt(1, 16)  ParameterScaling=2^0  OutDataType=fixdt(1, 16)  OutScaling=2^0
  int : Outport
  wires:
  Gain2/1 -> Add/2
  Gain3/1 -> Add/3
  byte0/1 -> Add/1
  Add/1 -> int/1
  byte1/1 -> Gain2/1
  byte2/1 -> Gain3/1
  byte3/1 -> Gain4/1
  Gain4/1 -> Add/4

== system Sim_Forcing_003h_expe_infra5_full_control2/BEC (May 7, 2015)/CAN Receive/Convert 4*uni8 to int3 ==
  byte0 : Inport
  byte1 : Inport  Port=2
  byte2 : Inport  Port=3
  byte3 : Inport  Port=4
  Add : Sum  Inputs=++++  OutDataTypeMode=int32  OutDataType=fixdt(1, 16)  OutScaling=2^-10  OutDataTypeStr=int32
  Gain2 : Gain  Gain=256  ParameterDataType=fixdt(1, 16)  ParameterScaling=2^0  OutDataType=fixdt(1, 16)  OutScaling=2^0
  Gain3 : Gain  Gain=2^16  ParameterDataType=fixdt(1, 16)  ParameterScaling=2^0  OutDataType=fixdt(1, 16)  OutScaling=2^0
  Gain4 : Gain  Gain=2^24  ParameterDataType=fixdt(1, 16)  ParameterScaling=2^0  OutDataType=fixdt(1, 16)  OutScaling=2^0
  int : Outport
  wires:
  Gain4/1 -> Add/4
  byte3/1 -> Gain4/1
  byte2/1 -> Gain3/1
  byte1/1 -> Gain2/1
  Add/1 -> int/1
  byte0/1 -> Add/1
  Gain3/1 -> Add/3
  Gain2/1 -> Add/2

== system Sim_Forcing_003h_expe_infra5_full_control2/BEC (May 7, 2015)/CAN Receive/Convert 4*uni8 to int4 ==
  byte0 : Inport
  byte1 : Inport  Port=2
  byte2 : Inport  Port=3
  byte3 : Inport  Port=4
  Add : Sum  Inputs=++++  OutDataTypeMode=int32  OutDataType=fixdt(1, 16)  OutScaling=2^-10  OutDataTypeStr=int32
  Gain2 : Gain  Gain=256  ParameterDataType=fixdt(1, 16)  ParameterScaling=2^0  OutDataType=fixdt(1, 16)  OutScaling=2^0
  Gain3 : Gain  Gain=2^16  ParameterDataType=fixdt(1, 16)  ParameterScaling=2^0  OutDataType=fixdt(1, 16)  OutScaling=2^0
  Gain4 : Gain  Gain=2^24  ParameterDataType=fixdt(1, 16)  ParameterScaling=2^0  OutDataType=fixdt(1, 16)  OutScaling=2^0
  int : Outport
  wires:
  Gain2/1 -> Add/2
  Gain3/1 -> Add/3
  byte0/1 -> Add/1
  Add/1 -> int/1
  byte1/1 -> Gain2/1
  byte2/1 -> Gain3/1
  byte3/1 -> Gain4/1
  Gain4/1 -> Add/4

== system Sim_Forcing_003h_expe_infra5_full_control2/BEC (May 7, 2015)/CAN Receive/Convert 4*uni8 to int5 ==
  byte0 : Inport
  byte1 : Inport  Port=2
  byte2 : Inport  Port=3
  byte3 : Inport  Port=4
  Add : Sum  Inputs=++++  OutDataTypeMode=int32  OutDataType=fixdt(1, 16)  OutScaling=2^-10  OutDataTypeStr=int32
  Gain2 : Gain  Gain=256  ParameterDataType=fixdt(1, 16)  ParameterScaling=2^0  OutDataType=fixdt(1, 16)  OutScaling=2^0
  Gain3 : Gain  Gain=2^16  ParameterDataType=fixdt(1, 16)  ParameterScaling=2^0  OutDataType=fixdt(1, 16)  OutScaling=2^0
  Gain4 : Gain  Gain=2^24  ParameterDataType=fixdt(1, 16)  ParameterScaling=2^0  OutDataType=fixdt(1, 16)  OutScaling=2^0
  int : Outport
  wires:
  Gain4/1 -> Add/4
  byte3/1 -> Gain4/1
  byte2/1 -> Gain3/1
  byte1/1 -> Gain2/1
  Add/1 -> int/1
  byte0/1 -> Add/1
  Gain3/1 -> Add/3
  Gain2/1 -> Add/2

== system Sim_Forcing_003h_expe_infra5_full_control2/BEC (May 7, 2015)/CAN Send/If Action Subsystem1 ==
  In1 : Inport  OutDataType=fixdt(1, 16)  OutScaling=2^0
  In2 : Inport  Port=2  OutDataType=fixdt(1, 16)  OutScaling=2^0
  In3 : Inport  Port=3  OutDataType=fixdt(1, 16)  OutScaling=2^0
  In4 : Inport  Port=4  OutDataType=fixdt(1, 16)  OutScaling=2^0
  In5 : Inport  Port=5  OutDataType=fixdt(1, 16)  OutScaling=2^0
  In6 : Inport  Port=6  OutDataType=fixdt(1, 16)  OutScaling=2^0
  Action Port : ActionPort  ActionType=then
  "Convert int to 4*uni8 " : Subsystem
  Convert int to 4*uni8 1 : Subsystem
  Convert int to 4*uni8 2 : Subsystem
  Convert int to 4*uni8 3 : Subsystem
  Convert int to 4*uni8 4 : Subsystem
  Convert int to 4*uni8 5 : Subsystem
  GT-RT CAN TX : gt_rt_lib/GT-RT CAN TX  uri='gt_rt_dev://localhost/dev/can0#0'  mff=MFF_11_DAT
  GT-RT CAN TX1 : gt_rt_lib/GT-RT CAN TX  uri='gt_rt_dev://localhost/dev/can0#0'  mff=MFF_11_DAT
  GT-RT CAN TX2 : gt_rt_lib/GT-RT CAN TX  uri='gt_rt_dev://localhost/dev/can0#0'  mff=MFF_11_DAT
  Mux : Mux  Inputs=2
  Mux1 : Mux  Inputs=2
  Mux2 : Mux  Inputs=2
  TX CAN ID1 : Constant  Value=hex2dec('101')  OutDataTypeMode=uint32  OutDataType=sfix(16)  OutScaling=2^0  OutDataTypeStr=uint32
  TX CAN ID2 : Constant  Value=hex2dec('102')  OutDataTypeMode=uint32  OutDataType=sfix(16)  OutScaling=2^0  OutDataTypeStr=uint32
  TX CAN ID3 : Constant  Value=hex2dec('103')  OutDataTypeMode=uint32  OutDataType=sfix(16)  OutScaling=2^0  OutDataTypeStr=uint32
  wires:
  In1/1 -> "Convert int to 4*uni8 "/1(in)
  In2/1 -> Convert int to 4*uni8 1/1(in)
  In3/1 -> Convert int to 4*uni8 2/1(in)
  In4/1 -> Convert int to 4*uni8 3/1(in)
  In5/1 -> Convert int to 4*uni8 4/1(in)
  In6/1 -> Convert int to 4*uni8 5/1(in)
  Mux2/1 -> GT-RT CAN TX2/2
  Convert int to 4*uni8 5/1(out) -> Mux2/2
  Convert int to 4*uni8 4/1(out) -> Mux2/1
  Mux1/1 -> GT-RT CAN TX1/2
  Convert int to 4*uni8 3/1(out) -> Mux1/2
  Convert int to 4*uni8 2/1(out) -> Mux1/1
  Mux/1 -> GT-RT CAN TX/2
  Convert int to 4*uni8 1/1(out) -> Mux/2
  "Convert int to 4*uni8 "/1(out) -> Mux/1
  TX CAN ID3/1 -> GT-RT CAN TX2/1
  TX CAN ID2/1 -> GT-RT CAN TX1/1
  TX CAN ID1/1 -> GT-RT CAN TX/1

== system Sim_Forcing_003h_expe_infra5_full_control2/BEC (May 7, 2015)/Software limit switches/Subsystem ==
  In1 : Inport
  act : Inport  Port=2
  Abs1 : Abs  OutDataType=fixdt(1, 16)  OutScaling=2^0
  Abs2 : Abs  OutDataType=fixdt(1, 16)  OutScaling=2^0
  Add1 : Sum  Inputs=+-  OutDataType=fixdt(1, 16)  OutScaling=2^-10
  Add2 : Sum  Inputs=-+  OutDataType=fixdt(1, 16)  OutScaling=2^-10
  Display : Display
  Display2 : Display
  If Action Subsystem : Subsystem  TreatAsAtomicUnit=on
  If Action Subsystem1 : Subsystem  TreatAsAtomicUnit=on
  If2 : If
  NSEA1 : Constant  Value=-160  OutDataType=fixdt(1, 16)  OutScaling=2^0
  PSEA1 : Constant  Value=160  OutDataType=fixdt(1, 16)  OutScaling=2^0
  Switch : Switch  Criteria=u2 > Threshold  OutDataType=fixdt(1, 16)  OutScaling=2^0
  Switch1 : Switch  Criteria=u2 ~= 0  OutDataType=fixdt(1, 16)  OutScaling=2^0
  Out1 : Outport
  wires:
  If Action Subsystem1/1(Out1) -> Switch/3
  If Action Subsystem/1(Out1) -> Display/1, Switch/1
  Abs1/1 -> If Action Subsystem1/2(dif)
  If2/2 -> If Action Subsystem1/Action
  If2/1 -> If Action Subsystem/Action
  In1/1 -> If2/1, If Action Subsystem/2(Inc), If Action Subsystem1/1(Inc), Switch/2, Switch1/2, Switch1/3
  Abs2/1 -> If Action Subsystem/1(dif)
  NSEA1/1 -> Add1/2
  PSEA1/1 -> Add2/1
  Add1/1 -> Abs1/1
  Add2/1 -> Abs2/1
  Switch/1 -> Switch1/1
  Switch1/1 -> Out1/1, Display2/1
  act/1 -> Add1/1, Add2/2

== system Sim_Forcing_003h_expe_infra5_full_control2/BEC (May 7, 2015)/Software limit switches/Subsystem1 ==
  In1 : Inport
  act : Inport  Port=2
  Abs1 : Abs  OutDataType=fixdt(1, 16)  OutScaling=2^0
  Abs2 : Abs  OutDataType=fixdt(1, 16)  OutScaling=2^0
  Add1 : Sum  Inputs=+-  OutDataType=fixdt(1, 16)  OutScaling=2^-10
  Add2 : Sum  Inputs=-+  OutDataType=fixdt(1, 16)  OutScaling=2^-10
  If Action Subsystem : Subsystem  TreatAsAtomicUnit=on
  If Action Subsystem1 : Subsystem  TreatAsAtomicUnit=on
  If2 : If
  NSEA1 : Constant  Value=-130  OutDataType=fixdt(1, 16)  OutScaling=2^0
  PSEA1 : Constant  Value=20  OutDataType=fixdt(1, 16)  OutScaling=2^0
  Switch : Switch  OutDataType=fixdt(1, 16)  OutScaling=2^0
  Switch1 : Switch  Criteria=u2 ~= 0  OutDataType=fixdt(1, 16)  OutScaling=2^0
  Out1 : Outport
  wires:
  act/1 -> Add1/1, Add2/2
  Add2/1 -> Abs2/1
  Add1/1 -> Abs1/1
  PSEA1/1 -> Add2/1
  NSEA1/1 -> Add1/2
  Abs2/1 -> If Action Subsystem/1(dif)
  In1/1 -> If Action Subsystem1/1(Inc), If Action Subsystem/2(Inc), Switch/2, Switch1/2, Switch1/3, If2/1
  If2/1 -> If Action Subsystem/Action
  If2/2 -> If Action Subsystem1/Action
  Abs1/1 -> If Action Subsystem1/2(dif)
  If Action Subsystem/1(Out1) -> Switch/1
  If Action Subsystem1/1(Out1) -> Switch/3
  Switch/1 -> Switch1/1
  Switch1/1 -> Out1/1

== system Sim_Forcing_003h_expe_infra5_full_control2/BEC (May 7, 2015)/Software limit switches/Subsystem2 ==
  In1 : Inport
  act : Inport  Port=2
  Abs1 : Abs  OutDataType=fixdt(1, 16)  OutScaling=2^0
  Abs2 : Abs  OutDataType=fixdt(1, 16)  OutScaling=2^0
  Add1 : Sum  Inputs=+-  OutDataType=fixdt(1, 16)  OutScaling=2^-10
  Add2 : Sum  Inputs=-+  OutDataType=fixdt(1, 16)  OutScaling=2^-10
  If Action Subsystem : Subsystem  TreatAsAtomicUnit=on
  If Action Subsystem1 : Subsystem  TreatAsAtomicUnit=on
  If2 : If
  NSEA1 : Constant  Value=-88  OutDataType=fixdt(1, 16)  OutScaling=2^0
  PSEA1 : Constant  Value=88  OutDataType=fixdt(1, 16)  OutScaling=2^0
  Switch : Switch  OutDataType=fixdt(1, 16)  OutScaling=2^0
  Switch1 : Switch  Criteria=u2 ~= 0  OutDataType=fixdt(1, 16)  OutScaling=2^0
  Out1 : Outport
  wires:
  If Action Subsystem1/1(Out1) -> Switch/3
  If Action Subsystem/1(Out1) -> Switch/1
  Abs1/1 -> If Action Subsystem1/2(dif)
  If2/2 -> If Action Subsystem1/Action
  If2/1 -> If Action Subsystem/Action
  In1/1 -> If2/1, If Action Subsystem/2(Inc), If Action Subsystem1/1(Inc), Switch/2, Switch1/2, Switch1/3
  Abs2/1 -> If Action Subsystem/1(dif)
  NSEA1/1 -> Add1/2
  PSEA1/1 -> Add2/1
  Add1/1 -> Abs1/1
  Add2/1 -> Abs2/1
  act/1 -> Add1/1, Add2/2
  Switch/1 -> Switch1/1
  Switch1/1 -> Out1/1

== system Sim_Forcing_003h_expe_infra5_full_control2/BEC (May 7, 2015)/Software limit switches/Subsystem3 ==
  In1 : Inport
  act : Inport  Port=2
  Abs1 : Abs  OutDataType=fixdt(1, 16)  OutScaling=2^0
  Abs2 : Abs  OutDataType=fixdt(1, 16)  OutScaling=2^0
  Add1 : Sum  Inputs=+-  OutDataType=fixdt(1, 16)  OutScaling=2^-10
  Add2 : Sum  Inputs=-+  OutDataType=fixdt(1, 16)  OutScaling=2^-10
  If Action Subsystem : Subsystem  TreatAsAtomicUnit=on
  If Action Subsystem1 : Subsystem  TreatAsAtomicUnit=on
  If2 : If
  NSEA1 : Constant  Value=-350  OutDataType=fixdt(1, 16)  OutScaling=2^0
  PSEA1 : Constant  Value=350  OutDataType=fixdt(1, 16)  OutScaling=2^0
  Switch : Switch  OutDataType=fixdt(1, 16)  OutScaling=2^0
  Switch1 : Switch  Criteria=u2 ~= 0  OutDataType=fixdt(1, 16)  OutScaling=2^0
  Out1 : Outport
  wires:
  Add2/1 -> Abs2/1
  Add1/1 -> Abs1/1
  PSEA1/1 -> Add2/1
  NSEA1/1 -> Add1/2
  Abs2/1 -> If Action Subsystem/1(dif)
  In1/1 -> If Action Subsystem1/1(Inc), If Action Subsystem/2(Inc), Switch/2, Switch1/2, Switch1/3, If2/1
  If2/1 -> If Action Subsystem/Action
  If2/2 -> If Action Subsystem1/Action
  act/1 -> Add2/2, Add1/1
  Abs1/1 -> If Action Subsystem1/2(dif)
  If Action Subsystem/1(Out1) -> Switch/1
  If Action Subsystem1/1(Out1) -> Switch/3
  Switch/1 -> Switch1/1
  Switch1/1 -> Out1/1

== system Sim_Forcing_003h_expe_infra5_full_control2/BEC (May 7, 2015)/Software limit switches/Subsystem4 ==
  In1 : Inport
  act : Inport  Port=2
  Abs1 : Abs  OutDataType=fixdt(1, 16)  OutScaling=2^0
  Abs2 : Abs  OutDataType=fixdt(1, 16)  OutScaling=2^0
  Add1 : Sum  Inputs=+-  OutDataType=fixdt(1, 16)  OutScaling=2^-10
  Add2 : Sum  Inputs=-+  OutDataType=fixdt(1, 16)  OutScaling=2^-10
  If Action Subsystem : Subsystem  TreatAsAtomicUnit=on
  If Action Subsystem1 : Subsystem  TreatAsAtomicUnit=on
  If2 : If
  NSEA1 : Constant  Value=-61  OutDataType=fixdt(1, 16)  OutScaling=2^0
  PSEA1 : Constant  Value=61  OutDataType=fixdt(1, 16)  OutScaling=2^0
  Switch : Switch  OutDataType=fixdt(1, 16)  OutScaling=2^0
  Switch1 : Switch  Criteria=u2 ~= 0  OutDataType=fixdt(1, 16)  OutScaling=2^0
  Out1 : Outport
  wires:
  If Action Subsystem/1(Out1) -> Switch/1
  Abs1/1 -> If Action Subsystem1/2(dif)
  If2/2 -> If Action Subsystem1/Action
  If2/1 -> If Action Subsystem/Action
  In1/1 -> If2/1, If Action Subsystem/2(Inc), If Action Subsystem1/1(Inc), Switch/2, Switch1/2, Switch1/3
  Abs2/1 -> If Action Subsystem/1(dif)
  NSEA1/1 -> Add1/2
  PSEA1/1 -> Add2/1
  Add1/1 -> Abs1/1
  Add2/1 -> Abs2/1
  If Action Subsystem1/1(Out1) -> Switch/3
  Switch/1 -> Switch1/1
  Switch1/1 -> Out1/1
  act/1 -> Add2/2, Add1/1

== system Sim_Forcing_003h_expe_infra5_full_control2/BEC (May 7, 2015)/Software limit switches/Subsystem5 ==
  In1 : Inport
  act : Inport  Port=2
  Abs1 : Abs  OutDataType=fixdt(1, 16)  OutScaling=2^0
  Abs2 : Abs  OutDataType=fixdt(1, 16)  OutScaling=2^0
  Add1 : Sum  Inputs=+-  OutDataType=fixdt(1, 16)  OutScaling=2^-10
  Add2 : Sum  Inputs=-+  OutDataType=fixdt(1, 16)  OutScaling=2^-10
  If Action Subsystem : Subsystem  TreatAsAtomicUnit=on
  If Action Subsystem1 : Subsystem  TreatAsAtomicUnit=on
  If2 : If
  NSEA1 : Constant  Value=-350  OutDataType=fixdt(1, 16)  OutScaling=2^0
  PSEA1 : Constant  Value=350  OutDataType=fixdt(1, 16)  OutScaling=2^0
  Switch : Switch  OutDataType=fixdt(1, 16)  OutScaling=2^0
  Switch1 : Switch  Criteria=u2 ~= 0  OutDataType=fixdt(1, 16)  OutScaling=2^0
  Out1 : Outport
  wires:
  Add2/1 -> Abs2/1
  Add1/1 -> Abs1/1
  PSEA1/1 -> Add2/1
  NSEA1/1 -> Add1/2
  Abs2/1 -> If Action Subsystem/1(dif)
  In1/1 -> If Action Subsystem1/1(Inc), If Action Subsystem/2(Inc), Switch/2, Switch1/2, Switch1/3, If2/1
  If2/1 -> If Action Subsystem/Action
  If2/2 -> If Action Subsystem1/Action
  Abs1/1 -> If Action Subsystem1/2(dif)
  If Action Subsystem/1(Out1) -> Switch/1
  If Action Subsystem1/1(Out1) -> Switch/3
  Switch/1 -> Switch1/1
  Switch1/1 -> Out1/1
  act/1 -> Add2/2, Add1/1

== system Sim_Forcing_003h_expe_infra5_full_control2/Breaking_Control 20/07/15/Move UP1/Smooth Displacement Second-Order Filter, zeta 0.8 ==
  Step IN Reset on  either : Inport
  T : Inport  Port=2  OutDataType=fixdt(1, 16)  OutScaling=2^0
  (zeta*T_transfer)/pi : Gain  Gain=0.8/pi  ParameterDataType=fixdt(1, 16)  ParameterScaling=2^0  OutDataType=fixdt(1, 16)  OutScaling=2^0
  4*zeta*pi : Gain  Gain=3.2*pi  ParameterDataType=fixdt(1, 16)  ParameterScaling=2^0  OutDataType=fixdt(1, 16)  OutScaling=2^0
  4*zeta*pi/T_transfer /s : DiscreteIntegrator  gainval=1  ExternalReset=either  InitialConditionSource=external  SampleTime=0.004  OutDataType=fixdt(1, 16)  OutScaling=2^0  ICPrevOutput=DiscIntNeverNeededParam  ICPrevScaledInput=DiscIntNeverNeededParam
  Discrete Derivative : simulink/Discrete/Discrete Derivative  SystemSampleTime=-1  gainval=1.0  ICPrevScaledInput=0.0  OutMin=[]  OutMax=[]  OutDataType=fixdt(1, 16)  OutScaling=2^-10  DoSatur=off
  Divide : Product  Inputs=*/  OutDataType=fixdt(1, 16)  OutScaling=2^-10
  Divide1 : Product  Inputs=*/  OutDataType=fixdt(1, 16)  OutScaling=2^-10
  For saving position  and velocity until after switchover : UnitDelay  SampleTime=-1
  Product : Product  OutDataType=fixdt(1, 16)  OutScaling=2^0  RndMeth=Zero
  Sum1 : Sum  Inputs=|+-  OutDataType=fixdt(1, 16)  OutScaling=2^0
  Sum2 : Sum  Inputs=-+|  OutDataType=fixdt(1, 16)  OutScaling=2^0
  pi/(zeta*T_transfer)/s : DiscreteIntegrator  gainval=1  ExternalReset=either  InitialConditionSource=external  SampleTime=0.004  OutDataType=fixdt(1, 16)  OutScaling=2^0  ICPrevOutput=DiscIntNeverNeededParam  ICPrevScaledInput=DiscIntNeverNeededParam
  pi/zeta : Gain  Gain=pi/0.8  ParameterDataType=fixdt(1, 16)  ParameterScaling=2^0  OutDataType=fixdt(1, 16)  OutScaling=2^0
  Out : Outport
  wires:
  Discrete Derivative/1 -> Product/2
  Product/1 -> (zeta*T_transfer)/pi/1
  Divide/1 -> 4*zeta*pi/1
  Divide1/1 -> pi/zeta/1
  pi/zeta/1 -> pi/(zeta*T_transfer)/s/1
  pi/(zeta*T_transfer)/s/1 -> Sum2/1, Out/1, For saving position  and velocity until after switchover/1
  4*zeta*pi/T_transfer /s/1 -> Divide1/1, Sum1/2
  Sum1/1 -> Divide/1
  4*zeta*pi/1 -> 4*zeta*pi/T_transfer /s/1
  T/1 -> [T]
  Step IN Reset on  either/1 -> [Step], Sum2/2
  [Step] -> 4*zeta*pi/T_transfer /s/2
  [Step] -> pi/(zeta*T_transfer)/s/2
  [T] -> Divide/2
  For saving position  and velocity until after switchover/1 -> Discrete Derivative/1, pi/(zeta*T_transfer)/s/3
  [T] -> Product/1
  (zeta*T_transfer)/pi/1 -> 4*zeta*pi/T_transfer /s/3
  [T] -> Divide1/2
  Sum2/1 -> Sum1/1

== system Sim_Forcing_003h_expe_infra5_full_control2/Breaking_Control 20/07/15/Move UP1/add x_offset ==
  x_offset : Inport
  set_in : Inport  Port=2
  Embedded MATLAB Function : Stateflow chart
  set_out : Outport
  wires:
  x_offset/1 -> Embedded MATLAB Function/1(dx)
  Embedded MATLAB Function/1(set_out) -> set_out/1
  set_in/1 -> Embedded MATLAB Function/2(set_in)

== system Sim_Forcing_003h_expe_infra5_full_control2/Breaking_Control 20/07/15/Move_cabin/Rate Control Dynamics Phi ==
  Turn_rate_roll (deg/sec) : Inport
  reset : Inport  Port=2
  adjust_angle : Inport  Port=3
  start_x : Inport  Port=4
  reset from_connect_y : Inport  Port=5
  Constant : Constant  Value=0.1  OutDataType=fixdt(1, 16)  OutScaling=2^0
  Constant2 : Constant  Value=3  OutDataType=fixdt(1, 16)  OutScaling=2^0
  Discrete-Time Integrator1 : DiscreteIntegrator  ExternalReset=either  SampleTime=0.004  OutDataType=fixdt(1, 16)  OutScaling=2^0  ICPrevOutput=DiscIntNeverNeededParam  ICPrevScaledInput=DiscIntNeverNeededParam
  Limit to 5 : Saturate  UpperLimit=5  LowerLimit=-5  OutDataType=fixdt(1, 16)  OutScaling=2^0
  Logical Operator1 : Logic  AllPortsSameDT=off  OutDataTypeMode=boolean  LogicDataType=fixdt(0, 8)  OutDataTypeStr=boolean
  Logical Operator2 : Logic  Operator=OR  AllPortsSameDT=off  OutDataTypeMode=boolean  LogicDataType=fixdt(0, 8)  OutDataTypeStr=boolean
  Product : Product  OutDataType=fixdt(1, 16)  OutScaling=2^0  RndMeth=Zero
  "Second-Order Filter, zeta 0.8" : Subsystem
  "Smooth Displacement Second-Order Filter, zeta 0.8" : Subsystem
  phi (deg) : Outport
  phi_dot (deg/sec) : Outport  Port=2
  wires:
  Turn_rate_roll (deg/sec)/1 -> "Second-Order Filter, zeta 0.8"/1(u)
  "Second-Order Filter, zeta 0.8"/1(x) -> Limit to 5/1
  Constant/1 -> "Second-Order Filter, zeta 0.8"/2(T)
  Discrete-Time Integrator1/1 -> Product/1
  Product/1 -> phi (deg)/1
  "Smooth Displacement Second-Order Filter, zeta 0.8"/1(Out) -> Product/2
  Constant2/1 -> "Smooth Displacement Second-Order Filter, zeta 0.8"/2(T)
  Limit to 5/1 -> Discrete-Time Integrator1/1, phi_dot (deg/sec)/1
  adjust_angle/1 -> Logical Operator1/1
  start_x/1 -> Logical Operator1/2
  reset from_connect_y/1 -> Logical Operator2/2
  Logical Operator2/1 -> Discrete-Time Integrator1/2
  reset/1 -> Logical Operator2/1
  Logical Operator1/1 -> "Smooth Displacement Second-Order Filter, zeta 0.8"/1(Step IN Reset on  either)

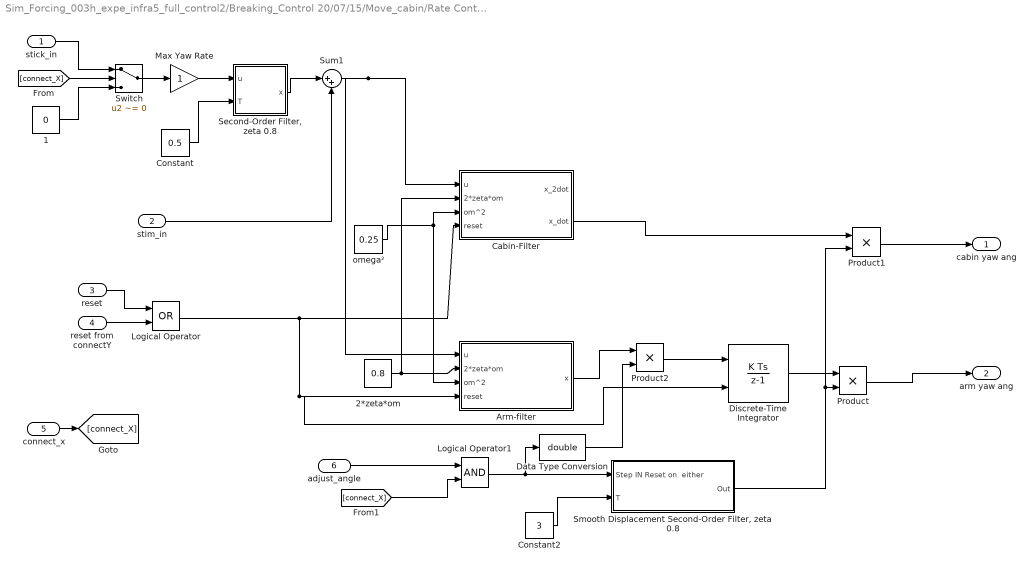
== system Sim_Forcing_003h_expe_infra5_full_control2/Breaking_Control 20/07/15/Move_cabin/Rate Control Dynamics Psi ==
  stick_in : Inport  OutDataType=fixdt(1, 16)  OutScaling=2^0
  stim_in : Inport  Port=2  OutDataType=fixdt(1, 16)  OutScaling=2^0
  reset : Inport  Port=3  OutDataType=fixdt(1, 16)  OutScaling=2^0
  reset from connectY : Inport  Port=4  OutDataType=fixdt(1, 16)  OutScaling=2^0
  connect_x : Inport  Port=5
  adjust_angle : Inport  Port=6
  1 : Constant  Value=0
  2*zeta*om : Constant  Value=0.8
  Arm-filter : Subsystem
  Cabin-Filter : Subsystem
  Constant : Constant  Value=0.5  OutDataType=fixdt(1, 16)  OutScaling=2^0
  Constant2 : Constant  Value=3  OutDataType=fixdt(1, 16)  OutScaling=2^0
  Data Type Conversion : DataTypeConversion  OutDataTypeMode=double  OutDataType=fixdt(1, 16)  OutScaling=2^0  OutDataTypeStr=double
  Discrete-Time Integrator : DiscreteIntegrator  ExternalReset=either  SampleTime=0.004  ICPrevOutput=DiscIntNeverNeededParam  ICPrevScaledInput=DiscIntNeverNeededParam
  Logical Operator : Logic  Operator=OR  AllPortsSameDT=off  OutDataTypeMode=boolean  LogicDataType=fixdt(0, 8)  OutDataTypeStr=boolean
  Logical Operator1 : Logic  AllPortsSameDT=off  OutDataTypeMode=boolean  LogicDataType=fixdt(0, 8)  OutDataTypeStr=boolean
  Max Yaw Rate : Gain
  Product : Product  OutDataType=fixdt(1, 16)  OutScaling=2^0  RndMeth=Zero
  Product1 : Product  OutDataType=fixdt(1, 16)  OutScaling=2^0  RndMeth=Zero
  Product2 : Product  OutDataType=fixdt(1, 16)  OutScaling=2^0  RndMeth=Zero
  "Second-Order Filter, zeta 0.8" : Subsystem
  "Smooth Displacement Second-Order Filter, zeta 0.8" : Subsystem
  Sum1 : Sum  Inputs=|++  OutDataType=fixdt(1, 16)  OutScaling=2^0
  Switch : Switch  Criteria=u2 ~= 0  OutDataType=fixdt(1, 16)  OutScaling=2^0
  omega² : Constant  Value=0.25
  cabin yaw ang : Outport  OutDataType=fixdt(1, 16)  OutScaling=2^0
  arm yaw ang : Outport  Port=2  OutDataType=fixdt(1, 16)  OutScaling=2^0
  wires:
  Sum1/1 -> Cabin-Filter/1(u), Arm-filter/1(u)
  stim_in/1 -> Sum1/2
  omega²/1 -> Arm-filter/3(om^2), Cabin-Filter/3(om^2)
  2*zeta*om/1 -> Arm-filter/2(2*zeta*om), Cabin-Filter/2(2*zeta*om)
  reset from connectY/1 -> Logical Operator/2
  reset/1 -> Logical Operator/1
  Logical Operator/1 -> Cabin-Filter/4(reset), Arm-filter/4(reset), Discrete-Time Integrator/2
  stick_in/1 -> Switch/1
  Switch/1 -> Max Yaw Rate/1
  1/1 -> Switch/3
  Constant2/1 -> "Smooth Displacement Second-Order Filter, zeta 0.8"/2(T)
  adjust_angle/1 -> Logical Operator1/1
  Logical Operator1/1 -> "Smooth Displacement Second-Order Filter, zeta 0.8"/1(Step IN Reset on  either), Data Type Conversion/1
  Discrete-Time Integrator/1 -> Product/1
  Product/1 -> arm yaw ang/1
  "Smooth Displacement Second-Order Filter, zeta 0.8"/1(Out) -> Product/2, Product1/2
  Cabin-Filter/2(x_dot) -> Product1/1
  Product1/1 -> cabin yaw ang/1
  connect_x/1 -> [connect_X]
  [connect_X] -> Switch/2
  [connect_X] -> Logical Operator1/2
  Arm-filter/1(x) -> Product2/1
  Product2/1 -> Discrete-Time Integrator/1
  Data Type Conversion/1 -> Product2/2
  Constant/1 -> "Second-Order Filter, zeta 0.8"/2(T)
  Max Yaw Rate/1 -> "Second-Order Filter, zeta 0.8"/1(u)
  "Second-Order Filter, zeta 0.8"/1(x) -> Sum1/1

== system Sim_Forcing_003h_expe_infra5_full_control2/Breaking_Control 20/07/15/Move_cabin/Rate Control Dynamics Theta ==
  Turn_rate_pitch (deg/sec) : Inport
  reset : Inport  Port=2
  adjust_angle : Inport  Port=3
  start_x : Inport  Port=4
  reset from_connect_y : Inport  Port=5
  Constant : Constant  Value=0.1  OutDataType=fixdt(1, 16)  OutScaling=2^0
  Constant2 : Constant  Value=3  OutDataType=fixdt(1, 16)  OutScaling=2^0
  Discrete-Time Integrator1 : DiscreteIntegrator  ExternalReset=either  SampleTime=0.004  OutDataType=fixdt(1, 16)  OutScaling=2^0  ICPrevOutput=DiscIntNeverNeededParam  ICPrevScaledInput=DiscIntNeverNeededParam
  Limit to 5 : Saturate  UpperLimit=5  LowerLimit=-5  OutDataType=fixdt(1, 16)  OutScaling=2^0
  Logical Operator1 : Logic  AllPortsSameDT=off  OutDataTypeMode=boolean  LogicDataType=fixdt(0, 8)  OutDataTypeStr=boolean
  Logical Operator2 : Logic  Operator=OR  AllPortsSameDT=off  OutDataTypeMode=boolean  LogicDataType=fixdt(0, 8)  OutDataTypeStr=boolean
  Product : Product  OutDataType=fixdt(1, 16)  OutScaling=2^0  RndMeth=Zero
  "Second-Order Filter, zeta 0.8" : Subsystem
  "Smooth Displacement Second-Order Filter, zeta 0.8" : Subsystem
  theta (deg) : Outport
  theta_dot (deg/sec) : Outport  Port=2
  wires:
  Turn_rate_pitch (deg/sec)/1 -> "Second-Order Filter, zeta 0.8"/1(u)
  "Second-Order Filter, zeta 0.8"/1(x) -> Limit to 5/1
  Constant/1 -> "Second-Order Filter, zeta 0.8"/2(T)
  Discrete-Time Integrator1/1 -> Product/1
  Product/1 -> theta (deg)/1
  "Smooth Displacement Second-Order Filter, zeta 0.8"/1(Out) -> Product/2
  Constant2/1 -> "Smooth Displacement Second-Order Filter, zeta 0.8"/2(T)
  Limit to 5/1 -> Discrete-Time Integrator1/1, theta_dot (deg/sec)/1
  Logical Operator1/1 -> "Smooth Displacement Second-Order Filter, zeta 0.8"/1(Step IN Reset on  either)
  adjust_angle/1 -> Logical Operator1/1
  start_x/1 -> Logical Operator1/2
  reset/1 -> Logical Operator2/1
  reset from_connect_y/1 -> Logical Operator2/2
  Logical Operator2/1 -> Discrete-Time Integrator1/2
